simulink model "Glider_FTA"  (Simulink 8.0)
settings: Solver=ode45  StartTime=0.0  StopTime=20000  RelTol=1e-3
settings Model: Creator=KOO  LastModifiedBy=KOO

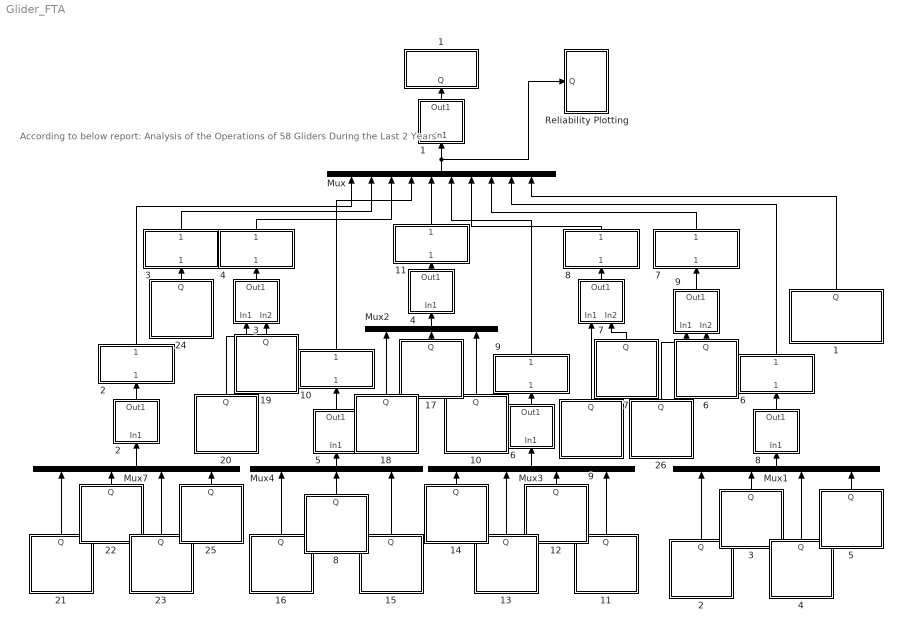
== system Glider_FTA ==
  note: According to below report:
      | Analysis of the Operations of 58 Gliders During the Last 2 Years
  "   1" : Subsystem
      mask Display:
      | % Use engine icon for subsystem
      | image(imread('OR.jpg'))
      | % Basic Event Name
      | fprintf('OR')
  "   2" : Subsystem
      mask Display:
      | % Use engine icon for subsystem
      | image(imread('OR.jpg'))
      | % Basic Event Name
      | fprintf('OR')
  "   3" : Subsystem
      mask Display:
      | % Use engine icon for subsystem
      | image(imread('OR.jpg'))
      | % Basic Event Name
      | fprintf('OR')
  "   4" : Subsystem
      mask Display:
      | % Use engine icon for subsystem
      | image(imread('OR.jpg'))
      | % Basic Event Name
      | fprintf('OR')
  "   5" : Subsystem
      mask Display:
      | % Use engine icon for subsystem
      | image(imread('OR.jpg'))
      | % Basic Event Name
      | fprintf('OR')
  "   6" : Subsystem
      mask Display:
      | % Use engine icon for subsystem
      | image(imread('OR.jpg'))
      | % Basic Event Name
      | fprintf('OR')
  "   7" : Subsystem
      mask Display:
      | % Use engine icon for subsystem
      | image(imread('OR.jpg'))
      | % Basic Event Name
      | fprintf('OR')
  "   8" : Subsystem
      mask Display:
      | % Use engine icon for subsystem
      | image(imread('OR.jpg'))
      | % Basic Event Name
      | fprintf('OR')
  "   9" : Subsystem
      mask Display:
      | % Use engine icon for subsystem
      | image(imread('OR.jpg'))
      | % Basic Event Name
      | fprintf('OR')
  "           1" : Subsystem
      mask Display:
      | % Use engine icon for subsystem
      | image(imread('TOP.jpg'))
      | % Basic Event Name
      | fprintf('TOP')
  "           10" : Subsystem
      mask Display:
      | % Use engine icon for subsystem
      | image(imread('TOP.jpg'))
      | % Basic Event Name
      | fprintf('Environment\nDetection')
  "           11" : Subsystem
      mask Display:
      | % Use engine icon for subsystem
      | image(imread('TOP.jpg'))
      | % Basic Event Name
      | fprintf('Collision')
  "           2" : Subsystem
      mask Display:
      | % Use engine icon for subsystem
      | image(imread('TOP.jpg'))
      | % Basic Event Name
      | fprintf('Power')
  "           3" : Subsystem
      mask Display:
      | % Use engine icon for subsystem
      | image(imread('TOP.jpg'))
      | % Basic Event Name
      | fprintf('Leak')
  "           4" : Subsystem
      mask Display:
      | % Use engine icon for subsystem
      | image(imread('TOP.jpg'))
      | % Basic Event Name
      | fprintf('Diving')
  "           6" : Subsystem
      mask Display:
      | % Use engine icon for subsystem
      | image(imread('TOP.jpg'))
      | % Basic Event Name
      | fprintf('Navigation')
  "           7" : Subsystem
      mask Display:
      | % Use engine icon for subsystem
      | image(imread('TOP.jpg'))
      | % Basic Event Name
      | fprintf('Communication')
  "           8" : Subsystem
      mask Display:
      | % Use engine icon for subsystem
      | image(imread('TOP.jpg'))
      | % Basic Event Name
      | fprintf('Propultion')
  "           9" : Subsystem
      mask Display:
      | % Use engine icon for subsystem
      | image(imread('TOP.jpg'))
      | % Basic Event Name
      | fprintf('Computer')
  " 1" : Subsystem
      mask Display:
      | % Use engine icon for subsystem
      | image(imread('Tr.jpg'))
      | % Basic Event Name
      | fprintf('\nX25:\nUnknown')
  " 10" : Subsystem
      mask Display:
      | % Use engine icon for subsystem
      | image(imread('Basic.jpg'))
      | % Basic Event Name
      | fprintf('X17:\nGlider\nRecovered')
  " 11" : Subsystem
      mask Display:
      | % Use engine icon for subsystem
      | image(imread('Basic.jpg'))
      | % Basic Event Name
      | fprintf('X16:\nOnBoard\nSoftware')
  " 12" : Subsystem
      mask Display:
      | % Use engine icon for subsystem
      | image(imread('Basic.jpg'))
      | % Basic Event Name
      | fprintf('X15:\nCMD\nControl')
  " 13" : Subsystem
      mask Display:
      | % Use engine icon for subsystem
      | image(imread('Basic.jpg'))
      | % Basic Event Name
      | fprintf('X14:\nAttitude\nControl')
  " 14" : Subsystem
      mask Display:
      | % Use engine icon for subsystem
      | image(imread('Basic.jpg'))
      | % Basic Event Name
      | fprintf('X13:\nData\nLogging')
  " 15" : Subsystem
      mask Display:
      | % Use engine icon for subsystem
      | image(imread('Basic.jpg'))
      | % Basic Event Name
      | fprintf('X12:\nIridium\nComms')
  " 16" : Subsystem
      mask Display:
      | % Use engine icon for subsystem
      | image(imread('Basic.jpg'))
      | % Basic Event Name
      | fprintf('X10:\nScience\nSensor')
  " 17" : Subsystem
      mask Display:
      | % Use engine icon for subsystem
      | image(imread('Basic.jpg'))
      | % Basic Event Name
      | fprintf('X9:\nCollision\nSeabed')
  " 18" : Subsystem
      mask Display:
      | % Use engine icon for subsystem
      | image(imread('Basic.jpg'))
      | % Basic Event Name
      | fprintf('X8:\nCollision\nVessel')
  " 19" : Subsystem
      mask Display:
      | % Use engine icon for subsystem
      | image(imread('Basic.jpg'))
      | % Basic Event Name
      | fprintf('X7:\nAir Bladder\nLeak')
  " 2" : Subsystem
      mask Display:
      | % Use engine icon for subsystem
      | image(imread('Basic.jpg'))
      | % Basic Event Name
      | fprintf('X21\nGPS Host')
  " 20" : Subsystem
      mask Display:
      | % Use engine icon for subsystem
      | image(imread('Basic.jpg'))
      | % Basic Event Name
      | fprintf('X6:\nBuoyancy\nPump')
  " 21" : Subsystem
      mask Display:
      | % Use engine icon for subsystem
      | image(imread('Basic.jpg'))
      | % Basic Event Name
      | fprintf('X5:\nBattery\nDetection')
  " 22" : Subsystem
      mask Display:
      | % Use engine icon for subsystem
      | image(imread('Basic.jpg'))
      | % Basic Event Name
      | fprintf('X4:\nBattery')
  " 23" : Subsystem
      mask Display:
      | % Use engine icon for subsystem
      | image(imread('Basic.jpg'))
      | % Basic Event Name
      | fprintf('X3:\nVoltage\nDetection')
  " 24" : Subsystem
      mask Display:
      | % Use engine icon for subsystem
      | image(imread('Basic.jpg'))
      | % Basic Event Name
      | fprintf('X2:\nLeak\nDetection')
  " 25" : Subsystem
      mask Display:
      | % Use engine icon for subsystem
      | image(imread('Basic.jpg'))
      | % Basic Event Name
      | fprintf('X1:\nCurrent\nMonitoring')
  " 26" : Subsystem
      mask Display:
      | % Use engine icon for subsystem
      | image(imread('Basic.jpg'))
      | % Basic Event Name
      | fprintf('X12:\nIridium\nComm')
  " 3" : Subsystem
      mask Display:
      | % Use engine icon for subsystem
      | image(imread('Basic.jpg'))
      | % Basic Event Name
      | fprintf('X22:\nBAD GPS')
  " 4" : Subsystem
      mask Display:
      | % Use engine icon for subsystem
      | image(imread('Basic.jpg'))
      | % Basic Event Name
      | fprintf('X23:\nDigifin')
  " 5" : Subsystem
      mask Display:
      | % Use engine icon for subsystem
      | image(imread('Basic.jpg'))
      | % Basic Event Name
      | fprintf('X24:\nRoll Motor')
  " 6" : Subsystem
      mask Display:
      | % Use engine icon for subsystem
      | image(imread('Basic.jpg'))
      | % Basic Event Name
      | fprintf('X20:\nArgos')
  " 7" : Subsystem
      mask Display:
      | % Use engine icon for subsystem
      | image(imread('Basic.jpg'))
      | % Basic Event Name
      | fprintf('X19:\nFin Lock')
  " 8" : Subsystem
      mask Display:
      | % Use engine icon for subsystem
      | image(imread('Basic.jpg'))
      | % Basic Event Name
      | fprintf('X11:\nCTD')
  " 9" : Subsystem
      mask Display:
      | % Use engine icon for subsystem
      | image(imread('Basic.jpg'))
      | % Basic Event Name
      | fprintf('X18:\nRudder\nBroken')
  Mux : Mux  Inputs=10
  Mux1 : Mux
  Mux2 : Mux  Inputs=3
  Mux3 : Mux
  Mux4 : Mux  Inputs=3
  Mux7 : Mux
  Reliability Plotting : Subsystem
  wires:
  "   1"/1(Out1) -> "           1"/1(Q)
  Mux/1 -> "   1"/1(In1), Reliability Plotting/1(Q)
  " 5"/1(Q) -> Mux1/4
  " 4"/1(Q) -> Mux1/3
  " 3"/1(Q) -> Mux1/2
  " 2"/1(Q) -> Mux1/1
  " 7"/1(Q) -> "   7"/2(In2)
  " 9"/1(Q) -> "   7"/1(In1)
  "   7"/1(Out1) -> "           8"/1("  ")
  " 10"/1(Q) -> Mux2/3
  " 11"/1(Q) -> Mux3/4
  " 12"/1(Q) -> Mux3/3
  " 13"/1(Q) -> Mux3/2
  " 14"/1(Q) -> Mux3/1
  " 15"/1(Q) -> Mux4/3
  " 8"/1(Q) -> Mux4/2
  " 16"/1(Q) -> Mux4/1
  "   4"/1(Out1) -> "           11"/1("  ")
  " 17"/1(Q) -> Mux2/2
  "   3"/1(Out1) -> "           4"/1("  ")
  " 19"/1(Q) -> "   3"/2(In2)
  " 20"/1(Q) -> "   3"/1(In1)
  " 24"/1(Q) -> "           3"/1("  ")
  " 25"/1(Q) -> Mux7/4
  " 21"/1(Q) -> Mux7/1
  " 22"/1(Q) -> Mux7/2
  " 23"/1(Q) -> Mux7/3
  " 1"/1(Q) -> Mux/10
  "           6"/1("   ") -> Mux/9
  "           7"/1("   ") -> Mux/8
  "           8"/1("   ") -> Mux/7
  "           9"/1("   ") -> Mux/6
  "           4"/1("   ") -> Mux/3
  "           3"/1("   ") -> Mux/2
  "           2"/1("   ") -> Mux/1
  Mux7/1 -> "   2"/1(In1)
  "   2"/1(Out1) -> "           2"/1("  ")
  " 18"/1(Q) -> Mux2/1
  Mux4/1 -> "   5"/1(In1)
  "   5"/1(Out1) -> "           10"/1("  ")
  Mux3/1 -> "   6"/1(In1)
  "   6"/1(Out1) -> "           9"/1("  ")
  Mux1/1 -> "   8"/1(In1)
  "   8"/1(Out1) -> "           6"/1("  ")
  "           11"/1("   ") -> Mux/5
  "           10"/1("   ") -> Mux/4
  Mux2/1 -> "   4"/1(In1)
  "   9"/1(Out1) -> "           7"/1("  ")
  " 6"/1(Q) -> "   9"/2(In2)
  " 26"/1(Q) -> "   9"/1(In1)

== system Glider_FTA/   1 ==
  In1 : Inport
  Demux : Demux  Outputs=10
  MATLAB Function : MATLAB Function  TreatAsAtomicUnit=on
  Out1 : Outport
  wires:
  Demux/2 -> MATLAB Function/2(u2)
  MATLAB Function/1(y) -> Out1/1
  In1/1 -> Demux/1
  Demux/1 -> MATLAB Function/1(u1)
  Demux/3 -> MATLAB Function/3(u3)
  Demux/4 -> MATLAB Function/4(u4)
  Demux/5 -> MATLAB Function/5(u5)
  Demux/6 -> MATLAB Function/6(u6)
  Demux/7 -> MATLAB Function/7(u7)
  Demux/8 -> MATLAB Function/8(u8)
  Demux/9 -> MATLAB Function/9(u9)
  Demux/10 -> MATLAB Function/10(u10)

== system Glider_FTA/   2 ==
  In1 : Inport
  Demux : Demux
  MATLAB Function : MATLAB Function  TreatAsAtomicUnit=on
  Out1 : Outport
  wires:
  Demux/4 -> MATLAB Function/4(u4)
  Demux/3 -> MATLAB Function/3(u3)
  Demux/1 -> MATLAB Function/1(u1)
  In1/1 -> Demux/1
  MATLAB Function/1(y) -> Out1/1
  Demux/2 -> MATLAB Function/2(u2)

== system Glider_FTA/   3 ==
  In1 : Inport
  In2 : Inport  Port=2
  MATLAB Function : MATLAB Function  TreatAsAtomicUnit=on
  Out1 : Outport
  wires:
  MATLAB Function/1(y) -> Out1/1
  In2/1 -> MATLAB Function/2(u2)
  In1/1 -> MATLAB Function/1(u1)

== system Glider_FTA/   4 ==
  In1 : Inport
  Demux : Demux  Outputs=3
  MATLAB Function : MATLAB Function  TreatAsAtomicUnit=on
  Out1 : Outport
  wires:
  Demux/3 -> MATLAB Function/3(u3)
  Demux/1 -> MATLAB Function/1(u1)
  In1/1 -> Demux/1
  MATLAB Function/1(y) -> Out1/1
  Demux/2 -> MATLAB Function/2(u2)

== system Glider_FTA/   5 ==
  In1 : Inport
  Demux : Demux  Outputs=3
  MATLAB Function : MATLAB Function  TreatAsAtomicUnit=on
  Out1 : Outport
  wires:
  Demux/2 -> MATLAB Function/2(u2)
  MATLAB Function/1(y) -> Out1/1
  In1/1 -> Demux/1
  Demux/1 -> MATLAB Function/1(u1)
  Demux/3 -> MATLAB Function/3(u3)

== system Glider_FTA/   6 ==
  In1 : Inport
  Demux : Demux
  MATLAB Function : MATLAB Function  TreatAsAtomicUnit=on
  Out1 : Outport
  wires:
  Demux/4 -> MATLAB Function/4(u4)
  Demux/3 -> MATLAB Function/3(u3)
  Demux/1 -> MATLAB Function/1(u1)
  In1/1 -> Demux/1
  MATLAB Function/1(y) -> Out1/1
  Demux/2 -> MATLAB Function/2(u2)

== system Glider_FTA/   7 ==
  In1 : Inport
  In2 : Inport  Port=2
  MATLAB Function : MATLAB Function  TreatAsAtomicUnit=on
  Out1 : Outport
  wires:
  MATLAB Function/1(y) -> Out1/1
  In2/1 -> MATLAB Function/2(u2)
  In1/1 -> MATLAB Function/1(u1)

== system Glider_FTA/   8 ==
  In1 : Inport
  Demux : Demux
  MATLAB Function : MATLAB Function  TreatAsAtomicUnit=on
  Out1 : Outport
  wires:
  Demux/2 -> MATLAB Function/2(u2)
  MATLAB Function/1(y) -> Out1/1
  In1/1 -> Demux/1
  Demux/1 -> MATLAB Function/1(u1)
  Demux/3 -> MATLAB Function/3(u3)
  Demux/4 -> MATLAB Function/4(u4)

== system Glider_FTA/   9 ==
  In1 : Inport
  In2 : Inport  Port=2
  MATLAB Function : MATLAB Function  TreatAsAtomicUnit=on
  Out1 : Outport
  wires:
  In1/1 -> MATLAB Function/1(u1)
  In2/1 -> MATLAB Function/2(u2)
  MATLAB Function/1(y) -> Out1/1

== system Glider_FTA/           1 ==
  Q : Inport
  1 : Constant
  Sum1 : Sum  Inputs=|+-
  Total Reliability : Scope
      settings: SaveName=Y
  wires:
  Q/1 -> Sum1/2
  Sum1/1 -> Total Reliability/1
  1/1 -> Sum1/1

== system Glider_FTA/           10 ==
  "  " : Inport
  "   " : Outport
  wires:
  "  "/1 -> "   "/1

== system Glider_FTA/           11 ==
  "  " : Inport
  "   " : Outport
  wires:
  "  "/1 -> "   "/1

== system Glider_FTA/           2 ==
  "  " : Inport
  "   " : Outport
  wires:
  "  "/1 -> "   "/1

== system Glider_FTA/           3 ==
  "  " : Inport
  "   " : Outport
  wires:
  "  "/1 -> "   "/1

== system Glider_FTA/           4 ==
  "  " : Inport
  "   " : Outport
  wires:
  "  "/1 -> "   "/1

== system Glider_FTA/           6 ==
  "  " : Inport
  "   " : Outport
  wires:
  "  "/1 -> "   "/1

== system Glider_FTA/           7 ==
  "  " : Inport
  "   " : Outport
  wires:
  "  "/1 -> "   "/1

== system Glider_FTA/           8 ==
  "  " : Inport
  "   " : Outport
  wires:
  "  "/1 -> "   "/1

== system Glider_FTA/           9 ==
  "  " : Inport
  "   " : Outport
  wires:
  "  "/1 -> "   "/1

== system Glider_FTA/ 1 ==
  Landa : Constant  Value=3.624*10^-6
  Time_Exp1 : Subsystem
  Q : Outport
  wires:
  Landa/1 -> Time_Exp1/1(Landa)
  Time_Exp1/1(Q) -> Q/1

== system Glider_FTA/ 10 ==
  Landa : Constant  Value=1.812*10^-6
  Time_Exp1 : Subsystem
  Q : Outport
  wires:
  Time_Exp1/1(Q) -> Q/1
  Landa/1 -> Time_Exp1/1(Landa)

== system Glider_FTA/ 11 ==
  Landa : Constant  Value=0.908*10^-6
  Time_Exp1 : Subsystem
  Q : Outport
  wires:
  Landa/1 -> Time_Exp1/1(Landa)
  Time_Exp1/1(Q) -> Q/1

== system Glider_FTA/ 12 ==
  Landa : Constant  Value=0.908*10^-6
  Time_Exp1 : Subsystem
  Q : Outport
  wires:
  Time_Exp1/1(Q) -> Q/1
  Landa/1 -> Time_Exp1/1(Landa)

== system Glider_FTA/ 13 ==
  Landa : Constant  Value=2.719*10^-6
  Time_Exp1 : Subsystem
  Q : Outport
  wires:
  Landa/1 -> Time_Exp1/1(Landa)
  Time_Exp1/1(Q) -> Q/1

== system Glider_FTA/ 14 ==
  Landa : Constant  Value=1.812*10^-6
  Time_Exp1 : Subsystem
  Q : Outport
  wires:
  Time_Exp1/1(Q) -> Q/1
  Landa/1 -> Time_Exp1/1(Landa)

== system Glider_FTA/ 15 ==
  Landa : Constant  Value=3.624*10^-6
  Time_Exp1 : Subsystem
  Q : Outport
  wires:
  Landa/1 -> Time_Exp1/1(Landa)
  Time_Exp1/1(Q) -> Q/1

== system Glider_FTA/ 16 ==
  Landa : Constant  Value=3.624*10^-6
  Time_Exp1 : Subsystem
  Q : Outport
  wires:
  Time_Exp1/1(Q) -> Q/1
  Landa/1 -> Time_Exp1/1(Landa)

== system Glider_FTA/ 17 ==
  Landa : Constant  Value=1.812*10^-6
  Time_Exp1 : Subsystem
  Q : Outport
  wires:
  Landa/1 -> Time_Exp1/1(Landa)
  Time_Exp1/1(Q) -> Q/1

== system Glider_FTA/ 18 ==
  Landa : Constant  Value=3.624*10^-6
  Time_Exp1 : Subsystem
  Q : Outport
  wires:
  Time_Exp1/1(Q) -> Q/1
  Landa/1 -> Time_Exp1/1(Landa)

== system Glider_FTA/ 19 ==
  Landa : Constant  Value=0.908*10^-6
  Time_Exp1 : Subsystem
  Q : Outport
  wires:
  Landa/1 -> Time_Exp1/1(Landa)
  Time_Exp1/1(Q) -> Q/1

== system Glider_FTA/ 2 ==
  Landa : Constant  Value=8.5*10^-6
  Time_Exp1 : Subsystem
  Q : Outport
  wires:
  Landa/1 -> Time_Exp1/1(Landa)
  Time_Exp1/1(Q) -> Q/1

== system Glider_FTA/ 20 ==
  Landa : Constant  Value=5.436*10^-6
  Time_Exp1 : Subsystem
  Q : Outport
  wires:
  Time_Exp1/1(Q) -> Q/1
  Landa/1 -> Time_Exp1/1(Landa)

== system Glider_FTA/ 21 ==
  Landa : Constant  Value=7.5*10^-6
  Time_Exp1 : Subsystem
  Q : Outport
  wires:
  Landa/1 -> Time_Exp1/1(Landa)
  Time_Exp1/1(Q) -> Q/1

== system Glider_FTA/ 22 ==
  Landa : Constant  Value=8.154*10^-6
  Time_Exp1 : Subsystem
  Q : Outport
  wires:
  Time_Exp1/1(Q) -> Q/1
  Landa/1 -> Time_Exp1/1(Landa)

== system Glider_FTA/ 23 ==
  Landa : Constant  Value=6.5*10^-6
  Time_Exp1 : Subsystem
  Q : Outport
  wires:
  Landa/1 -> Time_Exp1/1(Landa)
  Time_Exp1/1(Q) -> Q/1

== system Glider_FTA/ 24 ==
  Landa : Constant  Value=13.59*10^-6
  Time_Exp1 : Subsystem
  Q : Outport
  wires:
  Time_Exp1/1(Q) -> Q/1
  Landa/1 -> Time_Exp1/1(Landa)

== system Glider_FTA/ 25 ==
  Landa : Constant  Value=6.5*10^-6
  Time_Exp1 : Subsystem
  Q : Outport
  wires:
  Landa/1 -> Time_Exp1/1(Landa)
  Time_Exp1/1(Q) -> Q/1

== system Glider_FTA/ 26 ==
  Landa : Constant  Value=3.624*10^-6
  Time_Exp1 : Subsystem
  Q : Outport
  wires:
  Time_Exp1/1(Q) -> Q/1
  Landa/1 -> Time_Exp1/1(Landa)

== system Glider_FTA/ 3 ==
  Landa : Constant  Value=13.413*10^-6
  Time_Exp1 : Subsystem
  Q : Outport
  wires:
  Landa/1 -> Time_Exp1/1(Landa)
  Time_Exp1/1(Q) -> Q/1

== system Glider_FTA/ 4 ==
  Landa : Constant  Value=0.908*10^-6
  Time_Exp1 : Subsystem
  Q : Outport
  wires:
  Time_Exp1/1(Q) -> Q/1
  Landa/1 -> Time_Exp1/1(Landa)

== system Glider_FTA/ 5 ==
  Landa : Constant  Value=0.908*10^-6
  Time_Exp1 : Subsystem
  Q : Outport
  wires:
  Landa/1 -> Time_Exp1/1(Landa)
  Time_Exp1/1(Q) -> Q/1

== system Glider_FTA/ 6 ==
  Landa : Constant  Value=0.908*10^-6
  Time_Exp1 : Subsystem
  Q : Outport
  wires:
  Landa/1 -> Time_Exp1/1(Landa)
  Time_Exp1/1(Q) -> Q/1

== system Glider_FTA/ 7 ==
  Landa : Constant  Value=0.908*10^-6
  Time_Exp1 : Subsystem
  Q : Outport
  wires:
  Time_Exp1/1(Q) -> Q/1
  Landa/1 -> Time_Exp1/1(Landa)

== system Glider_FTA/ 8 ==
  Landa : Constant  Value=.2*10^-6
  Time_Exp1 : Subsystem
  Q : Outport
  wires:
  Time_Exp1/1(Q) -> Q/1
  Landa/1 -> Time_Exp1/1(Landa)

== system Glider_FTA/ 9 ==
  Landa : Constant  Value=0.908*10^-6
  Time_Exp1 : Subsystem
  Q : Outport
  wires:
  Landa/1 -> Time_Exp1/1(Landa)
  Time_Exp1/1(Q) -> Q/1

== system Glider_FTA/Reliability Plotting ==
  Q : Inport
  1 : Constant
  Demux : Demux  Outputs=10
  Reliability : Scope  NumInputPorts=10
      settings: YMin=-5~-5~-5~-5~-5~-5~-5~-5~-5~-5  YMax=5~5~5~5~5~5~5~5~5~5  SaveName=Reliability
  Sum1 : Sum  Inputs=|+-
  wires:
  Sum1/1 -> Demux/1
  1/1 -> Sum1/1
  Demux/6 -> Reliability/6
  Demux/5 -> Reliability/5
  Demux/4 -> Reliability/4
  Demux/7 -> Reliability/7
  Demux/8 -> Reliability/8
  Demux/9 -> Reliability/9
  Demux/3 -> Reliability/3
  Demux/1 -> Reliability/1
  Demux/2 -> Reliability/2
  Q/1 -> Sum1/2
  Demux/10 -> Reliability/10

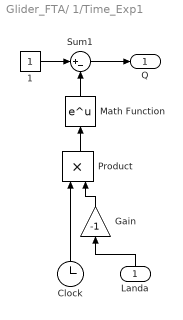
== system Glider_FTA/ 1/Time_Exp1 ==
  Landa : Inport
  1 : Constant
  Clock : Clock
  Gain : Gain  Gain=-1
  Math Function : Math  OutputSignalType=real  SaturateOnIntegerOverflow=on
  Product : Product  RndMeth=Zero
  Sum1 : Sum  Inputs=|+-
  Q : Outport
  wires:
  Landa/1 -> Gain/1
  Gain/1 -> Product/2
  Product/1 -> Math Function/1
  Clock/1 -> Product/1
  Math Function/1 -> Sum1/2
  1/1 -> Sum1/1
  Sum1/1 -> Q/1

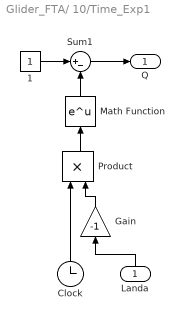
== system Glider_FTA/ 10/Time_Exp1 ==
  Landa : Inport
  1 : Constant
  Clock : Clock
  Gain : Gain  Gain=-1
  Math Function : Math  OutputSignalType=real  SaturateOnIntegerOverflow=on
  Product : Product  RndMeth=Zero
  Sum1 : Sum  Inputs=|+-
  Q : Outport
  wires:
  Sum1/1 -> Q/1
  1/1 -> Sum1/1
  Math Function/1 -> Sum1/2
  Clock/1 -> Product/1
  Product/1 -> Math Function/1
  Gain/1 -> Product/2
  Landa/1 -> Gain/1

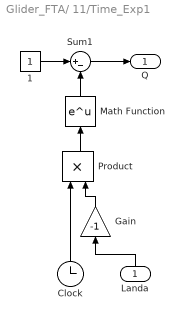
== system Glider_FTA/ 11/Time_Exp1 ==
  Landa : Inport
  1 : Constant
  Clock : Clock
  Gain : Gain  Gain=-1
  Math Function : Math  OutputSignalType=real  SaturateOnIntegerOverflow=on
  Product : Product  RndMeth=Zero
  Sum1 : Sum  Inputs=|+-
  Q : Outport
  wires:
  Landa/1 -> Gain/1
  Gain/1 -> Product/2
  Product/1 -> Math Function/1
  Clock/1 -> Product/1
  Math Function/1 -> Sum1/2
  1/1 -> Sum1/1
  Sum1/1 -> Q/1

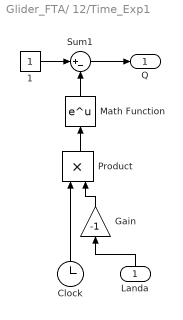
== system Glider_FTA/ 12/Time_Exp1 ==
  Landa : Inport
  1 : Constant
  Clock : Clock
  Gain : Gain  Gain=-1
  Math Function : Math  OutputSignalType=real  SaturateOnIntegerOverflow=on
  Product : Product  RndMeth=Zero
  Sum1 : Sum  Inputs=|+-
  Q : Outport
  wires:
  Sum1/1 -> Q/1
  1/1 -> Sum1/1
  Math Function/1 -> Sum1/2
  Clock/1 -> Product/1
  Product/1 -> Math Function/1
  Gain/1 -> Product/2
  Landa/1 -> Gain/1

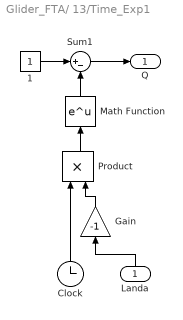
== system Glider_FTA/ 13/Time_Exp1 ==
  Landa : Inport
  1 : Constant
  Clock : Clock
  Gain : Gain  Gain=-1
  Math Function : Math  OutputSignalType=real  SaturateOnIntegerOverflow=on
  Product : Product  RndMeth=Zero
  Sum1 : Sum  Inputs=|+-
  Q : Outport
  wires:
  Landa/1 -> Gain/1
  Gain/1 -> Product/2
  Product/1 -> Math Function/1
  Clock/1 -> Product/1
  Math Function/1 -> Sum1/2
  1/1 -> Sum1/1
  Sum1/1 -> Q/1

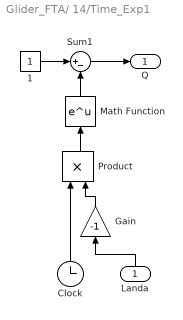
== system Glider_FTA/ 14/Time_Exp1 ==
  Landa : Inport
  1 : Constant
  Clock : Clock
  Gain : Gain  Gain=-1
  Math Function : Math  OutputSignalType=real  SaturateOnIntegerOverflow=on
  Product : Product  RndMeth=Zero
  Sum1 : Sum  Inputs=|+-
  Q : Outport
  wires:
  Sum1/1 -> Q/1
  1/1 -> Sum1/1
  Math Function/1 -> Sum1/2
  Clock/1 -> Product/1
  Product/1 -> Math Function/1
  Gain/1 -> Product/2
  Landa/1 -> Gain/1

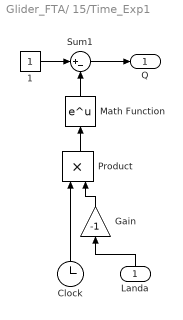
== system Glider_FTA/ 15/Time_Exp1 ==
  Landa : Inport
  1 : Constant
  Clock : Clock
  Gain : Gain  Gain=-1
  Math Function : Math  OutputSignalType=real  SaturateOnIntegerOverflow=on
  Product : Product  RndMeth=Zero
  Sum1 : Sum  Inputs=|+-
  Q : Outport
  wires:
  Landa/1 -> Gain/1
  Gain/1 -> Product/2
  Product/1 -> Math Function/1
  Clock/1 -> Product/1
  Math Function/1 -> Sum1/2
  1/1 -> Sum1/1
  Sum1/1 -> Q/1

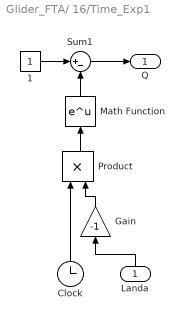
== system Glider_FTA/ 16/Time_Exp1 ==
  Landa : Inport
  1 : Constant
  Clock : Clock
  Gain : Gain  Gain=-1
  Math Function : Math  OutputSignalType=real  SaturateOnIntegerOverflow=on
  Product : Product  RndMeth=Zero
  Sum1 : Sum  Inputs=|+-
  Q : Outport
  wires:
  Sum1/1 -> Q/1
  1/1 -> Sum1/1
  Math Function/1 -> Sum1/2
  Clock/1 -> Product/1
  Product/1 -> Math Function/1
  Gain/1 -> Product/2
  Landa/1 -> Gain/1

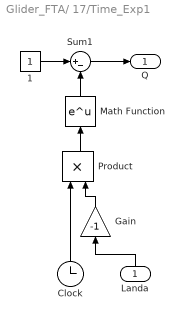
== system Glider_FTA/ 17/Time_Exp1 ==
  Landa : Inport
  1 : Constant
  Clock : Clock
  Gain : Gain  Gain=-1
  Math Function : Math  OutputSignalType=real  SaturateOnIntegerOverflow=on
  Product : Product  RndMeth=Zero
  Sum1 : Sum  Inputs=|+-
  Q : Outport
  wires:
  Landa/1 -> Gain/1
  Gain/1 -> Product/2
  Product/1 -> Math Function/1
  Clock/1 -> Product/1
  Math Function/1 -> Sum1/2
  1/1 -> Sum1/1
  Sum1/1 -> Q/1

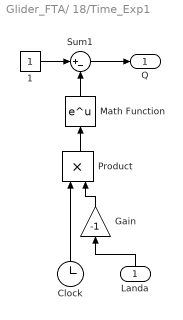
== system Glider_FTA/ 18/Time_Exp1 ==
  Landa : Inport
  1 : Constant
  Clock : Clock
  Gain : Gain  Gain=-1
  Math Function : Math  OutputSignalType=real  SaturateOnIntegerOverflow=on
  Product : Product  RndMeth=Zero
  Sum1 : Sum  Inputs=|+-
  Q : Outport
  wires:
  Sum1/1 -> Q/1
  1/1 -> Sum1/1
  Math Function/1 -> Sum1/2
  Clock/1 -> Product/1
  Product/1 -> Math Function/1
  Gain/1 -> Product/2
  Landa/1 -> Gain/1

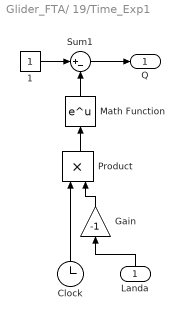
== system Glider_FTA/ 19/Time_Exp1 ==
  Landa : Inport
  1 : Constant
  Clock : Clock
  Gain : Gain  Gain=-1
  Math Function : Math  OutputSignalType=real  SaturateOnIntegerOverflow=on
  Product : Product  RndMeth=Zero
  Sum1 : Sum  Inputs=|+-
  Q : Outport
  wires:
  Landa/1 -> Gain/1
  Gain/1 -> Product/2
  Product/1 -> Math Function/1
  Clock/1 -> Product/1
  Math Function/1 -> Sum1/2
  1/1 -> Sum1/1
  Sum1/1 -> Q/1

== system Glider_FTA/ 2/Time_Exp1 ==
  Landa : Inport
  1 : Constant
  Clock : Clock
  Gain : Gain  Gain=-1
  Math Function : Math  OutputSignalType=real  SaturateOnIntegerOverflow=on
  Product : Product  RndMeth=Zero
  Sum1 : Sum  Inputs=|+-
  Q : Outport
  wires:
  Landa/1 -> Gain/1
  Gain/1 -> Product/2
  Product/1 -> Math Function/1
  Clock/1 -> Product/1
  Math Function/1 -> Sum1/2
  1/1 -> Sum1/1
  Sum1/1 -> Q/1

== system Glider_FTA/ 20/Time_Exp1 ==
  Landa : Inport
  1 : Constant
  Clock : Clock
  Gain : Gain  Gain=-1
  Math Function : Math  OutputSignalType=real  SaturateOnIntegerOverflow=on
  Product : Product  RndMeth=Zero
  Sum1 : Sum  Inputs=|+-
  Q : Outport
  wires:
  Sum1/1 -> Q/1
  1/1 -> Sum1/1
  Math Function/1 -> Sum1/2
  Clock/1 -> Product/1
  Product/1 -> Math Function/1
  Gain/1 -> Product/2
  Landa/1 -> Gain/1

== system Glider_FTA/ 21/Time_Exp1 ==
  Landa : Inport
  1 : Constant
  Clock : Clock
  Gain : Gain  Gain=-1
  Math Function : Math  OutputSignalType=real  SaturateOnIntegerOverflow=on
  Product : Product  RndMeth=Zero
  Sum1 : Sum  Inputs=|+-
  Q : Outport
  wires:
  Landa/1 -> Gain/1
  Gain/1 -> Product/2
  Product/1 -> Math Function/1
  Clock/1 -> Product/1
  Math Function/1 -> Sum1/2
  1/1 -> Sum1/1
  Sum1/1 -> Q/1

== system Glider_FTA/ 22/Time_Exp1 ==
  Landa : Inport
  1 : Constant
  Clock : Clock
  Gain : Gain  Gain=-1
  Math Function : Math  OutputSignalType=real  SaturateOnIntegerOverflow=on
  Product : Product  RndMeth=Zero
  Sum1 : Sum  Inputs=|+-
  Q : Outport
  wires:
  Sum1/1 -> Q/1
  1/1 -> Sum1/1
  Math Function/1 -> Sum1/2
  Clock/1 -> Product/1
  Product/1 -> Math Function/1
  Gain/1 -> Product/2
  Landa/1 -> Gain/1

== system Glider_FTA/ 23/Time_Exp1 ==
  Landa : Inport
  1 : Constant
  Clock : Clock
  Gain : Gain  Gain=-1
  Math Function : Math  OutputSignalType=real  SaturateOnIntegerOverflow=on
  Product : Product  RndMeth=Zero
  Sum1 : Sum  Inputs=|+-
  Q : Outport
  wires:
  Landa/1 -> Gain/1
  Gain/1 -> Product/2
  Product/1 -> Math Function/1
  Clock/1 -> Product/1
  Math Function/1 -> Sum1/2
  1/1 -> Sum1/1
  Sum1/1 -> Q/1

== system Glider_FTA/ 24/Time_Exp1 ==
  Landa : Inport
  1 : Constant
  Clock : Clock
  Gain : Gain  Gain=-1
  Math Function : Math  OutputSignalType=real  SaturateOnIntegerOverflow=on
  Product : Product  RndMeth=Zero
  Sum1 : Sum  Inputs=|+-
  Q : Outport
  wires:
  Sum1/1 -> Q/1
  1/1 -> Sum1/1
  Math Function/1 -> Sum1/2
  Clock/1 -> Product/1
  Product/1 -> Math Function/1
  Gain/1 -> Product/2
  Landa/1 -> Gain/1

== system Glider_FTA/ 25/Time_Exp1 ==
  Landa : Inport
  1 : Constant
  Clock : Clock
  Gain : Gain  Gain=-1
  Math Function : Math  OutputSignalType=real  SaturateOnIntegerOverflow=on
  Product : Product  RndMeth=Zero
  Sum1 : Sum  Inputs=|+-
  Q : Outport
  wires:
  Landa/1 -> Gain/1
  Gain/1 -> Product/2
  Product/1 -> Math Function/1
  Clock/1 -> Product/1
  Math Function/1 -> Sum1/2
  1/1 -> Sum1/1
  Sum1/1 -> Q/1

== system Glider_FTA/ 26/Time_Exp1 ==
  Landa : Inport
  1 : Constant
  Clock : Clock
  Gain : Gain  Gain=-1
  Math Function : Math  OutputSignalType=real  SaturateOnIntegerOverflow=on
  Product : Product  RndMeth=Zero
  Sum1 : Sum  Inputs=|+-
  Q : Outport
  wires:
  Sum1/1 -> Q/1
  1/1 -> Sum1/1
  Math Function/1 -> Sum1/2
  Clock/1 -> Product/1
  Product/1 -> Math Function/1
  Gain/1 -> Product/2
  Landa/1 -> Gain/1

== system Glider_FTA/ 3/Time_Exp1 ==
  Landa : Inport
  1 : Constant
  Clock : Clock
  Gain : Gain  Gain=-1
  Math Function : Math  OutputSignalType=real  SaturateOnIntegerOverflow=on
  Product : Product  RndMeth=Zero
  Sum1 : Sum  Inputs=|+-
  Q : Outport
  wires:
  Landa/1 -> Gain/1
  Gain/1 -> Product/2
  Product/1 -> Math Function/1
  Clock/1 -> Product/1
  Math Function/1 -> Sum1/2
  1/1 -> Sum1/1
  Sum1/1 -> Q/1

== system Glider_FTA/ 4/Time_Exp1 ==
  Landa : Inport
  1 : Constant
  Clock : Clock
  Gain : Gain  Gain=-1
  Math Function : Math  OutputSignalType=real  SaturateOnIntegerOverflow=on
  Product : Product  RndMeth=Zero
  Sum1 : Sum  Inputs=|+-
  Q : Outport
  wires:
  Sum1/1 -> Q/1
  1/1 -> Sum1/1
  Math Function/1 -> Sum1/2
  Clock/1 -> Product/1
  Product/1 -> Math Function/1
  Gain/1 -> Product/2
  Landa/1 -> Gain/1

== system Glider_FTA/ 5/Time_Exp1 ==
  Landa : Inport
  1 : Constant
  Clock : Clock
  Gain : Gain  Gain=-1
  Math Function : Math  OutputSignalType=real  SaturateOnIntegerOverflow=on
  Product : Product  RndMeth=Zero
  Sum1 : Sum  Inputs=|+-
  Q : Outport
  wires:
  Landa/1 -> Gain/1
  Gain/1 -> Product/2
  Product/1 -> Math Function/1
  Clock/1 -> Product/1
  Math Function/1 -> Sum1/2
  1/1 -> Sum1/1
  Sum1/1 -> Q/1

== system Glider_FTA/ 6/Time_Exp1 ==
  Landa : Inport
  1 : Constant
  Clock : Clock
  Gain : Gain  Gain=-1
  Math Function : Math  OutputSignalType=real  SaturateOnIntegerOverflow=on
  Product : Product  RndMeth=Zero
  Sum1 : Sum  Inputs=|+-
  Q : Outport
  wires:
  Landa/1 -> Gain/1
  Gain/1 -> Product/2
  Product/1 -> Math Function/1
  Clock/1 -> Product/1
  Math Function/1 -> Sum1/2
  1/1 -> Sum1/1
  Sum1/1 -> Q/1

== system Glider_FTA/ 7/Time_Exp1 ==
  Landa : Inport
  1 : Constant
  Clock : Clock
  Gain : Gain  Gain=-1
  Math Function : Math  OutputSignalType=real  SaturateOnIntegerOverflow=on
  Product : Product  RndMeth=Zero
  Sum1 : Sum  Inputs=|+-
  Q : Outport
  wires:
  Sum1/1 -> Q/1
  1/1 -> Sum1/1
  Math Function/1 -> Sum1/2
  Clock/1 -> Product/1
  Product/1 -> Math Function/1
  Gain/1 -> Product/2
  Landa/1 -> Gain/1

== system Glider_FTA/ 8/Time_Exp1 ==
  Landa : Inport
  1 : Constant
  Clock : Clock
  Gain : Gain  Gain=-1
  Math Function : Math  OutputSignalType=real  SaturateOnIntegerOverflow=on
  Product : Product  RndMeth=Zero
  Sum1 : Sum  Inputs=|+-
  Q : Outport
  wires:
  Sum1/1 -> Q/1
  1/1 -> Sum1/1
  Math Function/1 -> Sum1/2
  Clock/1 -> Product/1
  Product/1 -> Math Function/1
  Gain/1 -> Product/2
  Landa/1 -> Gain/1

== system Glider_FTA/ 9/Time_Exp1 ==
  Landa : Inport
  1 : Constant
  Clock : Clock
  Gain : Gain  Gain=-1
  Math Function : Math  OutputSignalType=real  SaturateOnIntegerOverflow=on
  Product : Product  RndMeth=Zero
  Sum1 : Sum  Inputs=|+-
  Q : Outport
  wires:
  Landa/1 -> Gain/1
  Gain/1 -> Product/2
  Product/1 -> Math Function/1
  Clock/1 -> Product/1
  Math Function/1 -> Sum1/2
  1/1 -> Sum1/1
  Sum1/1 -> Q/1

== matlab function  2/MATLAB Function ==
  data: u1 input double; y output double; u2 input double; u3 input double; u4 input double
function y = FTA_OR(u1,u2,u3,u4)
%OR
y=1-((1-(u1)).*(1-(u2)).*(1-(u3)).*(1-(u4)));

== matlab function  3/MATLAB Function ==
  data: u1 input double; y output double; u2 input double
function y = FTA_OR(u1,u2)
%OR
y=1-((1-(u1)).*(1-(u2)));

== matlab function  1/MATLAB Function ==
  data: u1 input double; y output double; u2 input double; u3 input double; u4 input double; u5 input double; u6 input double; u7 input double; u8 input double; u9 input double; u10 input double
function y = FTA_OR(u1,u2,u3,u4,u5,u6,u7,u8,u9,u10)
%OR
y=1-((1-(u1)).*(1-(u2)).*(1-(u3)).*(1-(u4)).*(1-(u5))...
     .*(1-(u6)).*(1-(u7)).*(1-(u8)).*(1-(u9)).*(1-(u10)));

== matlab function  4/MATLAB Function ==
  data: u1 input double; y output double; u2 input double; u3 input double
function y = FTA_OR(u1,u2,u3)
%OR
y=1-((1-(u1)).*(1-(u2)).*(1-(u3)));

== matlab function  5/MATLAB Function ==
  data: u1 input double; y output double; u2 input double; u3 input double
function y = FTA_OR(u1,u2,u3)
%OR
y=1-((1-(u1)).*(1-(u2)).*(1-(u3)));

== matlab function  6/MATLAB Function ==
  data: u1 input double; y output double; u2 input double; u3 input double; u4 input double
function y = FTA_OR(u1,u2,u3,u4)
%OR
y=1-((1-(u1)).*(1-(u2)).*(1-(u3)).*(1-(u4)));

== matlab function  7/MATLAB Function ==
  data: u1 input double; y output double; u2 input double
function y = FTA_OR(u1,u2)
%OR
y=1-((1-(u1)).*(1-(u2)));

== matlab function  8/MATLAB Function ==
  data: u1 input double; y output double; u2 input double; u3 input double; u4 input double
function y = FTA_OR(u1,u2,u3,u4)
%OR
y=1-((1-(u1)).*(1-(u2)).*(1-(u3)).*(1-(u4)));

== matlab function  9/MATLAB Function ==
  data: u1 input double; y output double; u2 input double
function y = FTA_OR(u1,u2)
%OR
y=1-((1-(u1)).*(1-(u2)));
